simulink model "mConfigSetRef"  (Simulink 7.7)
settings: configuration reference "cs" (kept outside this file)
settings Model: Creator=hungdang  LastModifiedBy=hungdang

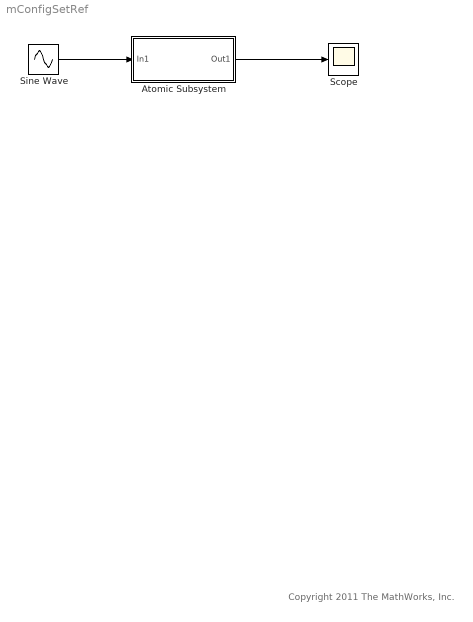
== system mConfigSetRef ==
  note: Copyright 2011 The MathWorks, Inc.
  Atomic Subsystem : Subsystem  TreatAsAtomicUnit=on
  Scope : Scope
  Sine Wave : Sin  SampleTime=0
  wires:
  Sine Wave/1 -> Atomic Subsystem/1(In1)
  Atomic Subsystem/1(Out1) -> Scope/1

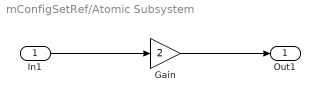
== system mConfigSetRef/Atomic Subsystem ==
  In1 : Inport
  Gain : Gain  Gain=2
  Out1 : Outport
  wires:
  In1/1 -> Gain/1
  Gain/1 -> Out1/1
